simulink model "openloop_test"  (R2023a)
settings: Solver=VariableStepAuto  StartTime=0.0  StopTime=10.0  RelTol=1e-3
libraries: cstblocks x2
settings Model: Creator=Yuganshu Wadhwa  LastModifiedBy=Yuganshu Wadhwa

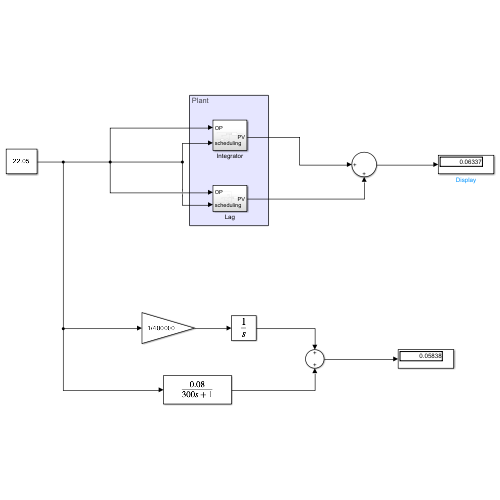
[thumbnail: Simulink's stored preview of the top-level diagram]
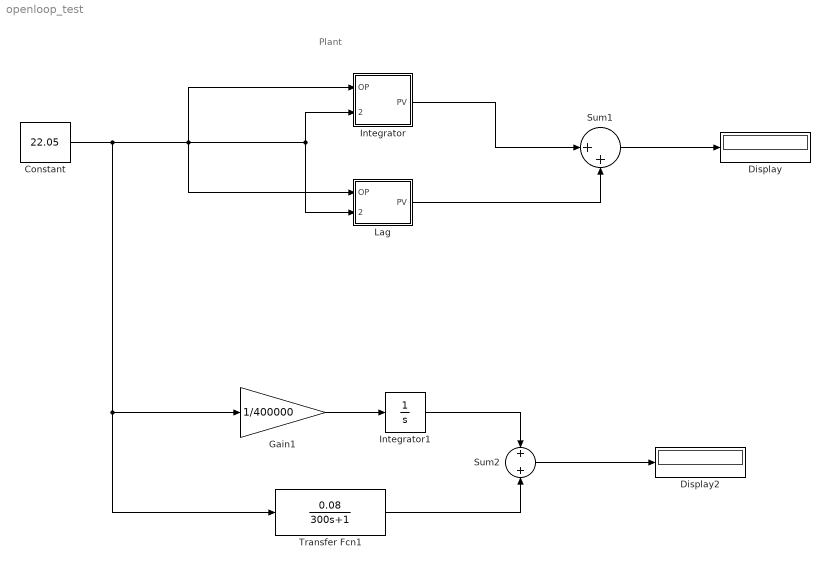
== system openloop_test ==
  note: Plant
  Constant : Constant  Value=22.05
  Display : Display
  Display2 : Display
  Gain1 : Gain  Gain=1/400000
  Integrator : Subsystem
  Integrator1 : Integrator
  Lag : Subsystem
  Sum1 : Sum  Inputs=|++
  Sum2 : Sum  Inputs=+|+
  Transfer Fcn1 : TransferFcn  Numerator=[0.08]  Denominator=|
      | [300
      |  1]
  wires:
  Integrator/1(PV) -> Sum1/1
  Lag/1(PV) -> Sum1/2
  Sum1/1 -> Display/1
  Constant/1 -> Lag/2(scheduling), Integrator/2(scheduling), Lag/1(OP), Integrator/1(OP), Gain1/1, Transfer Fcn1/1
  Transfer Fcn1/1 -> Sum2/2
  Gain1/1 -> Integrator1/1
  Integrator1/1 -> Sum2/1
  Sum2/1 -> Display2/1

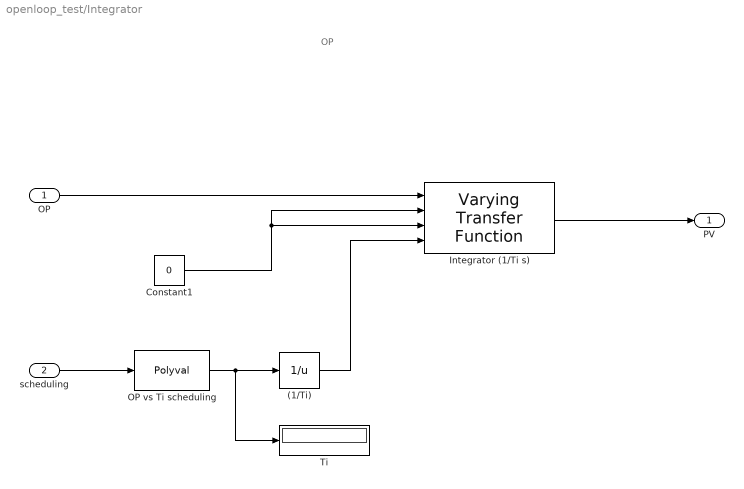
== system openloop_test/Integrator ==
  note: OP
  OP : Inport
  scheduling : Inport  Port=2
  (1/Ti) : Math  Operator=reciprocal
  Constant1 : Constant  Value=0
  Integrator (1/Ti s) : cstblocks/Linear Parameter Varying/Varying Transfer Function  N=1  Feedthrough=on
  OP vs Ti scheduling : Polyval  Coefs=[ +511.04, -14301, +405369 ]
  Ti : Display
  PV : Outport
  wires:
  OP/1 -> Integrator (1/Ti s)/1
  Constant1/1 -> Integrator (1/Ti s)/3, Integrator (1/Ti s)/2
  OP vs Ti scheduling/1 -> Ti/1, (1/Ti)/1
  Integrator (1/Ti s)/1 -> PV/1
  (1/Ti)/1 -> Integrator (1/Ti s)/4
  scheduling/1 -> OP vs Ti scheduling/1

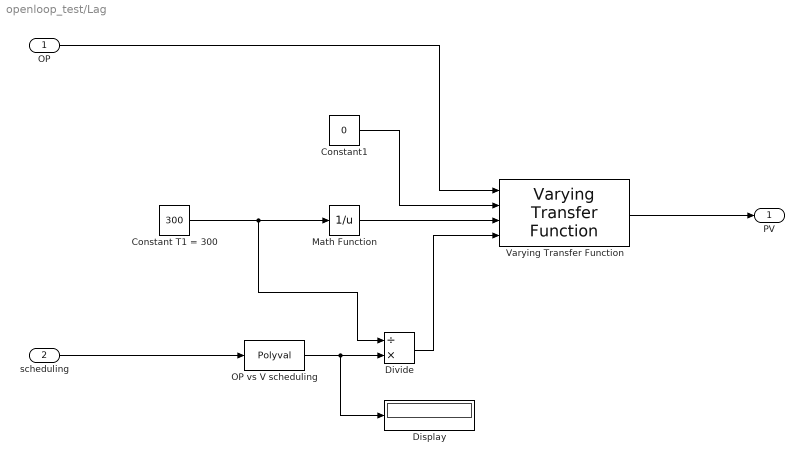
== system openloop_test/Lag ==
  OP : Inport
  scheduling : Inport  Port=2
  Constant T1 = 300 : Constant  Value=300
  Constant1 : Constant  Value=0
  Display : Display
  Divide : Product  Inputs=/*
  Math Function : Math  Operator=reciprocal
  OP vs V scheduling : Polyval  Coefs="[  -3e-7, +8e-5, -0.0065, 0.1944 ]"
  Varying Transfer Function : cstblocks/Linear Parameter Varying/Varying Transfer Function  N=1  Feedthrough=on
  PV : Outport
  wires:
  Divide/1 -> Varying Transfer Function/4
  Constant T1 = 300/1 -> Math Function/1, Divide/1
  Constant1/1 -> Varying Transfer Function/2
  OP/1 -> Varying Transfer Function/1
  OP vs V scheduling/1 -> Display/1, Divide/2
  Math Function/1 -> Varying Transfer Function/3
  Varying Transfer Function/1 -> PV/1
  scheduling/1 -> OP vs V scheduling/1
